simulink model "CDSC"  (R2018b)
settings: Solver=ode45  StartTime=0.0  StopTime=10.0  MaxStep=0.0001  MinStep=0.00001  RelTol=1e-3
libraries: simulink x1, powerlib_meascontrol x1, powerlib x1
settings Model: Creator=lokes  LastModifiedBy=lokes

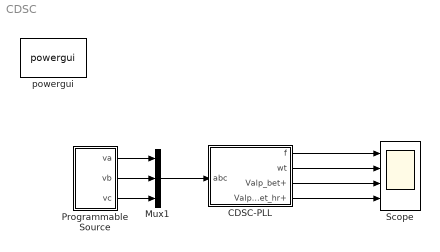
== system CDSC ==
  CDSC-PLL : Subsystem  mask{hr=7}
      mask prompts: hr "Required Component Extraction (hr)"
  Mux1 : Mux  Inputs=3
  Programmable Source : Subsystem  mask(CDSC - PLL){f=50, V=230}
      mask prompts: f "Fundamental grid frequency (f) in Hz"; V "Fundamental grid voltage (V) in RMS volts"
      mask help: Programmable source generates a signal with fundamental and odd harmonic signals upto 13th frequency component.
  Scope : Scope  NumInputPorts=4
  powergui : powerlib/powergui  Priority=1  SimulationMode=Discrete  SampleTime=10e-6  frequency=60  Iterations=50  frequencyindice=60  Pbase=100e6  ErrMax=1e-4  UnitsV=kV  UnitsW=MW  buscounter=0  FunctionMessages=off  echomessages=off  EnableUseOfTLC=off  CurrentSourceSwitches=off  DisableSnubberDevices=off  DisableRonSwitches=off  DisableVfSwitches=off  DisplayEquations=off  SolverType=Tustin/Backward Euler (TBE)  Interpol=off  ExternalGateDelay=off  methode=off  Ts=100  x0status=blocks  SPID=off  SwTol=0  HookPort=off  RestoreLinks=warning  ResistiveCurrentMeasurement=off  Frange=[0:2:500]  Ylog=off  Xlog=on  ShowGrid=off  save=off  variable=ZData  structure=0  ZoomFFT=off  StartTime=0.0  cycles=1  DisplayStyle=1  fundamental=60  FreqAxis=off  MaxFrequency=1000  frequencyindicesteady=1  RmsSteady=1  display=off
  wires:
  Mux1/1 -> CDSC-PLL/1(abc)
  Programmable Source/1(va) -> Mux1/1
  Programmable Source/2(vb) -> Mux1/2
  Programmable Source/3(vc) -> Mux1/3
  CDSC-PLL/1(f) -> Scope/1
  CDSC-PLL/2(wt) -> Scope/2
  CDSC-PLL/3(Valp_bet+) -> Scope/3
  CDSC-PLL/4(Valp_bet_hr+) -> Scope/4

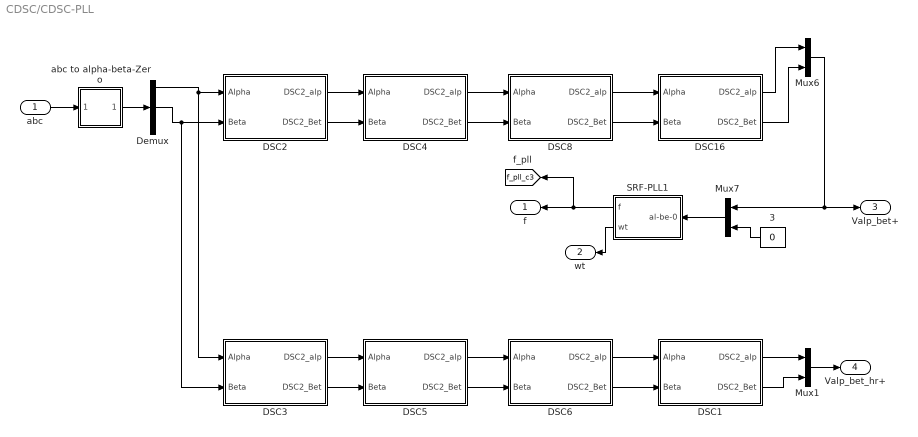
== system CDSC/CDSC-PLL ==
  abc : Inport
  3 : Constant  Value=0
  DSC1 : Subsystem  mask{n=16}
      mask prompts: n "DSC Number (n)"
  DSC16 : Subsystem  mask{n=16}
      mask prompts: n "DSC Number (n)"
  DSC2 : Subsystem  mask{n=2}
      mask prompts: n "DSC Number (n)"
  DSC3 : Subsystem  mask{n=2}
      mask prompts: n "DSC Number (n)"
  DSC4 : Subsystem  mask{n=4}
      mask prompts: n "DSC Number (n)"
  DSC5 : Subsystem  mask{n=4}
      mask prompts: n "DSC Number (n)"
  DSC6 : Subsystem  mask{n=8}
      mask prompts: n "DSC Number (n)"
  DSC8 : Subsystem  mask{n=8}
      mask prompts: n "DSC Number (n)"
  Demux : Demux  Outputs=3
  Mux1 : Mux  Inputs=2
  Mux6 : Mux  Inputs=2
  Mux7 : Mux  Inputs=2
  SRF-PLL1 : Subsystem
  abc to alpha-beta-Zero : Subsystem
      mask Display:
      | plot([0 1], [0,1])
      | text(0.15,0.7,'abc')
      | text(0.55, 0.3,'\alpha\beta0','texmode','on')
  f : Outport
  wt : Outport  Port=2
  Valp_bet+ : Outport  Port=3
  Valp_bet_hr+ : Outport  Port=4
  tag scope: f_pll_c3=global
  wires:
  abc/1 -> abc to alpha-beta-Zero/1(abc)
  abc to alpha-beta-Zero/1(al_be_0) -> Demux/1
  DSC2/1(DSC2_alp) -> DSC4/1(Alpha)
  DSC2/2(DSC2_Bet) -> DSC4/2(Beta)
  DSC4/1(DSC2_alp) -> DSC8/1(Alpha)
  DSC4/2(DSC2_Bet) -> DSC8/2(Beta)
  DSC8/1(DSC2_alp) -> DSC16/1(Alpha)
  DSC8/2(DSC2_Bet) -> DSC16/2(Beta)
  DSC16/1(DSC2_alp) -> Mux6/1
  DSC16/2(DSC2_Bet) -> Mux6/2
  Mux6/1 -> Valp_bet+/1, Mux7/1
  3/1 -> Mux7/2
  Mux7/1 -> SRF-PLL1/1(al-be-0)
  SRF-PLL1/1(f) -> [f_pll_c3], f/1
  SRF-PLL1/2(wt) -> wt/1
  Demux/1 -> DSC3/1(Alpha), DSC2/1(Alpha)
  Demux/2 -> DSC3/2(Beta), DSC2/2(Beta)
  DSC3/1(DSC2_alp) -> DSC5/1(Alpha)
  DSC3/2(DSC2_Bet) -> DSC5/2(Beta)
  DSC5/1(DSC2_alp) -> DSC6/1(Alpha)
  DSC5/2(DSC2_Bet) -> DSC6/2(Beta)
  DSC6/1(DSC2_alp) -> DSC1/1(Alpha)
  DSC6/2(DSC2_Bet) -> DSC1/2(Beta)
  DSC1/1(DSC2_alp) -> Mux1/1
  DSC1/2(DSC2_Bet) -> Mux1/2
  Mux1/1 -> Valp_bet_hr+/1

== system CDSC/Programmable Source ==
  1 : Sin  Amplitude=V*sqrt(2)  Frequency=2*pi*f  Phase=0*pi/2  SampleTime=0
  11 : Sin  Amplitude=V*sqrt(2)/11  Frequency=2*pi*11*f  Phase=0*pi/2  SampleTime=0
  13 : Sin  Amplitude=V*sqrt(2)/13  Frequency=2*pi*13*f  Phase=0*pi/2  SampleTime=0
  5 : Sin  Amplitude=V*sqrt(2)/5  Frequency=2*pi*5*f  Phase=0*pi/2  SampleTime=0
  7 : Sin  Amplitude=V*sqrt(2)/7  Frequency=2*pi*7*f  Phase=0*pi/2  SampleTime=0
  Constant : Constant  Value=2/(3*f)
  Constant1 : Constant  Value=1/(3*f)
  Gain : Gain
  Gain1 : Gain
  Gain2 : Gain
  Sum1 : Sum  Inputs=+++++
  Variable Transport Delay : VariableTransportDelay  VariableDelayType=Variable transport delay  MaximumDelay=10
  Variable Transport Delay1 : VariableTransportDelay  VariableDelayType=Variable transport delay  MaximumDelay=10
  va : Outport
  vb : Outport  Port=2
  vc : Outport  Port=3
  wires:
  Constant1/1 -> Variable Transport Delay1/2
  Constant/1 -> Variable Transport Delay/2
  Variable Transport Delay1/1 -> Gain/1
  Variable Transport Delay/1 -> Gain1/1
  Gain/1 -> vb/1
  Gain1/1 -> vc/1
  Sum1/1 -> Gain2/1
  Gain2/1 -> Variable Transport Delay1/1, Variable Transport Delay/1, va/1
  1/1 -> Sum1/1
  5/1 -> Sum1/2
  7/1 -> Sum1/3
  11/1 -> Sum1/4
  13/1 -> Sum1/5

== system CDSC/CDSC-PLL/DSC1 ==
  Alpha : Inport
  Beta : Inport  Port=2
  DSC_Beta : Subsystem
  DSC_alpha : Subsystem
  DSC2_alp : Outport
  DSC2_Bet : Outport  Port=2
  wires:
  Beta/1 -> DSC_Beta/2(Beta), DSC_alpha/2(Beta)
  Alpha/1 -> DSC_alpha/1(Alpha), DSC_Beta/1(Alpha)
  DSC_Beta/1(Out) -> DSC2_Bet/1
  DSC_alpha/1(Out) -> DSC2_alp/1

== system CDSC/CDSC-PLL/DSC16 ==
  Alpha : Inport
  Beta : Inport  Port=2
  DSC_Beta : Subsystem
  DSC_alpha : Subsystem
  DSC2_alp : Outport
  DSC2_Bet : Outport  Port=2
  wires:
  Beta/1 -> DSC_Beta/2(Beta), DSC_alpha/2(Beta)
  Alpha/1 -> DSC_alpha/1(Alpha), DSC_Beta/1(Alpha)
  DSC_Beta/1(Out) -> DSC2_Bet/1
  DSC_alpha/1(Out) -> DSC2_alp/1

== system CDSC/CDSC-PLL/DSC2 ==
  Alpha : Inport
  Beta : Inport  Port=2
  DSC_Beta : Subsystem
  DSC_alpha : Subsystem
  DSC2_alp : Outport
  DSC2_Bet : Outport  Port=2
  wires:
  DSC_alpha/1(Out) -> DSC2_alp/1
  DSC_Beta/1(Out) -> DSC2_Bet/1
  Alpha/1 -> DSC_Beta/1(Alpha), DSC_alpha/1(Alpha)
  Beta/1 -> DSC_alpha/2(Beta), DSC_Beta/2(Beta)

== system CDSC/CDSC-PLL/DSC3 ==
  Alpha : Inport
  Beta : Inport  Port=2
  DSC_Beta : Subsystem
  DSC_alpha : Subsystem
  DSC2_alp : Outport
  DSC2_Bet : Outport  Port=2
  wires:
  DSC_alpha/1(Out) -> DSC2_alp/1
  DSC_Beta/1(Out) -> DSC2_Bet/1
  Alpha/1 -> DSC_Beta/1(Alpha), DSC_alpha/1(Alpha)
  Beta/1 -> DSC_alpha/2(Beta), DSC_Beta/2(Beta)

== system CDSC/CDSC-PLL/DSC4 ==
  Alpha : Inport
  Beta : Inport  Port=2
  DSC_Beta : Subsystem
  DSC_alpha : Subsystem
  DSC2_alp : Outport
  DSC2_Bet : Outport  Port=2
  wires:
  Beta/1 -> DSC_Beta/2(Beta), DSC_alpha/2(Beta)
  Alpha/1 -> DSC_alpha/1(Alpha), DSC_Beta/1(Alpha)
  DSC_Beta/1(Out) -> DSC2_Bet/1
  DSC_alpha/1(Out) -> DSC2_alp/1

== system CDSC/CDSC-PLL/DSC5 ==
  Alpha : Inport
  Beta : Inport  Port=2
  DSC_Beta : Subsystem
  DSC_alpha : Subsystem
  DSC2_alp : Outport
  DSC2_Bet : Outport  Port=2
  wires:
  Beta/1 -> DSC_Beta/2(Beta), DSC_alpha/2(Beta)
  Alpha/1 -> DSC_alpha/1(Alpha), DSC_Beta/1(Alpha)
  DSC_Beta/1(Out) -> DSC2_Bet/1
  DSC_alpha/1(Out) -> DSC2_alp/1

== system CDSC/CDSC-PLL/DSC6 ==
  Alpha : Inport
  Beta : Inport  Port=2
  DSC_Beta : Subsystem
  DSC_alpha : Subsystem
  DSC2_alp : Outport
  DSC2_Bet : Outport  Port=2
  wires:
  DSC_alpha/1(Out) -> DSC2_alp/1
  DSC_Beta/1(Out) -> DSC2_Bet/1
  Alpha/1 -> DSC_Beta/1(Alpha), DSC_alpha/1(Alpha)
  Beta/1 -> DSC_alpha/2(Beta), DSC_Beta/2(Beta)

== system CDSC/CDSC-PLL/DSC8 ==
  Alpha : Inport
  Beta : Inport  Port=2
  DSC_Beta : Subsystem
  DSC_alpha : Subsystem
  DSC2_alp : Outport
  DSC2_Bet : Outport  Port=2
  wires:
  DSC_alpha/1(Out) -> DSC2_alp/1
  DSC_Beta/1(Out) -> DSC2_Bet/1
  Alpha/1 -> DSC_Beta/1(Alpha), DSC_alpha/1(Alpha)
  Beta/1 -> DSC_alpha/2(Beta), DSC_Beta/2(Beta)

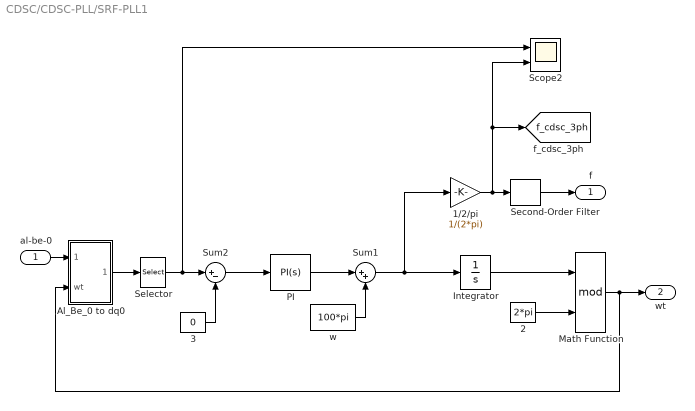
== system CDSC/CDSC-PLL/SRF-PLL1 ==
  al-be-0 : Inport
  1/2/pi : Gain  Gain=1/(2*pi)
  2 : Constant  Value=2*pi
  3 : Constant  Value=0
  Al_Be_0 to dq0 : Subsystem
      mask Display:
      | plot([0 1], [0,1])
      | port_label('input', 1, '\alpha\beta0','texmode','on')
      | port_label('input', 2, 'wt')
      | port_label('output', 1, 'dq0')
  Integrator : Integrator
  Math Function : Math  Operator=mod  SaturateOnIntegerOverflow=on
  "PI " : simulink/Continuous/PID Controller  Controller=PI  Form=Parallel  TimeDomain=Continuous-time  SampleTime=100e-6  IntegratorMethod=Forward Euler  FilterMethod=Forward Euler  ControllerParametersSource=internal  P=10  I=30  D=0  UseFilter=on  N=100  TunerSelectOption=Transfer Function Based (PID Tuner App)  InitialConditionSource=internal  InitialConditionForIntegrator=0  InitialConditionForFilter=0  DifferentiatorICPrevScaledInput=0  ExternalReset=none  TrackingMode=off  Kt=1  LimitOutput=off  UpperSaturationLimit=inf  LowerSaturationLimit=-inf  LinearizeAsGain=on  AntiWindupMode=none  Kb=1  POutMin=[]  POutMax=[]  IOutMin=[]  IOutMax=[]  DOutMin=[]  DOutMax=[]  NOutMin=[]  NOutMax=[]  SumOutMin=[]  SumOutMax=[]  SaturationOutMin=[]  SaturationOutMax=[]  PParamMin=[]  PParamMax=[]  IParamMin=[]  IParamMax=[]  DParamMin=[]  DParamMax=[]  NParamMin=[]  NParamMax=[]  KbParamMin=[]  KbParamMax=[]  KtParamMin=[]  KtParamMax=[]  KbOutMin=[]  KbOutMax=[]  KtOutMin=[]  KtOutMax=[]  IntegratorOutMin=[]  IntegratorOutMax=[]  FilterOutMin=[]  FilterOutMax=[]  SumI1OutMin=[]  SumI1OutMax=[]  SumI2OutMin=[]  SumI2OutMax=[]  SumI3OutMin=[]  SumI3OutMax=[]  SumI4OutMin=[]  SumI4OutMax=[]  SumDOutMin=[]  SumDOutMax=[]  DifferentiatorOutMin=[]  DifferentiatorOutMax=[]  FilterDiffOutCoefMin=[]  FilterDiffOutCoefMax=[]  ReciprocalOutMin=[]  ReciprocalOutMax=[]  SumDenOutMin=[]  SumDenOutMax=[]  SumNumOutMin=[]  SumNumOutMax=[]  DivideOutMin=[]  DivideOutMax=[]  IntegratorContinuousStateAttributes=''  IntegratorStateMustResolveToSignalObject=off  IntegratorRTWStateStorageClass=Auto  FilterContinuousStateAttributes=''  FilterStateMustResolveToSignalObject=off  FilterRTWStateStorageClass=Auto  ParallelPVariant=InternalParameters  IdealPVariant=Disabled  IVariant=InternalParameters  DVariant=Disabled  IntegratorVariant=Continuous  SatVariant=Disabled  AWVariant=Passthrough  PCopyVariant=Disabled  TRVariant=Disabled  FdbkBlocksVariant=Forward  IdealPFdbkVariant=Disabled  SatFdbkVariant=Disabled  DerivativeFilterVariant=Disabled  NVariant=Disabled  NCopyVariant=Disabled_SignalSpec  FilterICVariant=Disabled  IntegratorICVariant=InternalICs  ExternalResetVariant=Disabled  TRSumVariant=Passthrough  SumFdbkVariant=Disabled  SumVariant=Sum_PI
  Scope2 : Scope  NumInputPorts=2
  Second-Order Filter : powerlib_meascontrol/Filters/Second-Order Filter  FilterType=Lowpass  Fo=5  Zeta=0.707  Ts=0  Initialize=off  Vac_Init="[0,  0,  50]"  Vdc_Init=0  PlotResponse=off  FreqRange=[0, 500, 1]
      settings: SourceProductName=Simscape Electrical  SourceProductBaseCode=PS
  Selector : Selector  InputPortWidth=3  IndexOptions=Index vector (dialog)  Indices=1  OutputSizes=1
  Sum1 : Sum  Inputs=|++
  Sum2 : Sum  Inputs=|+-
  w : Constant  Value=100*pi
  f : Outport
  wt : Outport  Port=2
  tag scope: f_cdsc_3ph=global
  wires:
  1/2/pi/1 -> Second-Order Filter/1, [f_cdsc_3ph], Scope2/2
  Math Function/1 -> Al_Be_0 to dq0/2(wt), wt/1
  Integrator/1 -> Math Function/1
  2/1 -> Math Function/2
  Sum1/1 -> Integrator/1, 1/2/pi/1
  w/1 -> Sum1/2
  "PI "/1 -> Sum1/1
  Sum2/1 -> "PI "/1
  al-be-0/1 -> Al_Be_0 to dq0/1(Al_Be_0)
  3/1 -> Sum2/2
  Al_Be_0 to dq0/1(dq0) -> Selector/1
  Selector/1 -> Sum2/1, Scope2/1
  Second-Order Filter/1 -> f/1

== system CDSC/CDSC-PLL/abc to alpha-beta-Zero ==
  abc : Inport
  Gain1 : Gain  Gain=(2/3)  SaturateOnIntegerOverflow=on  OutDataTypeStr=Inherit: Same as input  ParamDataTypeStr=Inherit: Same as input
  Gain3 : Gain  Gain="[ 1   -1/2   -1/2; 0   sqrt(3)/2   -sqrt(3)/2; 1/(2)  1/(2)  1/(2) ]"  Multiplication=Matrix(K*u) (u vector)  SaturateOnIntegerOverflow=on  OutDataTypeStr=Inherit: Same as input  ParamDataTypeStr=Inherit: Same as input
  al_be_0 : Outport
  wires:
  Gain3/1 -> Gain1/1
  Gain1/1 -> al_be_0/1
  abc/1 -> Gain3/1

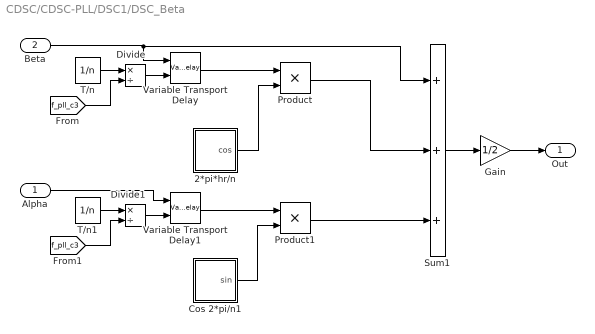
== system CDSC/CDSC-PLL/DSC1/DSC_Beta ==
  Alpha : Inport
  Beta : Inport  Port=2
  2*pi*hr/n : Subsystem
  Cos 2*pi/n1 : Subsystem
  Divide : Product  Inputs=*/
  Divide1 : Product  Inputs=*/
  Gain : Gain  Gain=1/2
  Product : Product
  Product1 : Product
  Sum1 : Sum  Inputs=+++
  T/n : Constant  Value=1/n
  T/n1 : Constant  Value=1/n
  Variable Transport Delay : VariableTransportDelay  VariableDelayType=Variable transport delay  MaximumDelay=10
  Variable Transport Delay1 : VariableTransportDelay  VariableDelayType=Variable transport delay  MaximumDelay=10
  Out : Outport
  wires:
  Gain/1 -> Out/1
  Sum1/1 -> Gain/1
  Beta/1 -> Variable Transport Delay/1, Sum1/1
  Alpha/1 -> Variable Transport Delay1/1
  2*pi*hr/n/1(cos) -> Product/2
  Product/1 -> Sum1/2
  Variable Transport Delay/1 -> Product/1
  Variable Transport Delay1/1 -> Product1/1
  Product1/1 -> Sum1/3
  Cos 2*pi/n1/1(sin) -> Product1/2
  T/n/1 -> Divide/1
  Divide/1 -> Variable Transport Delay/2
  [f_pll_c3] -> Divide/2
  T/n1/1 -> Divide1/1
  Divide1/1 -> Variable Transport Delay1/2
  [f_pll_c3] -> Divide1/2

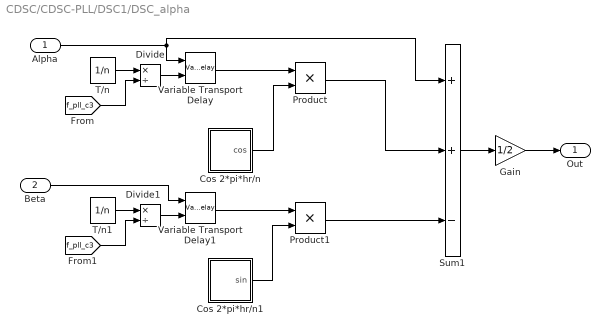
== system CDSC/CDSC-PLL/DSC1/DSC_alpha ==
  Alpha : Inport
  Beta : Inport  Port=2
  Cos 2*pi*hr/n : Subsystem
  Cos 2*pi*hr/n1 : Subsystem
  Divide : Product  Inputs=*/
  Divide1 : Product  Inputs=*/
  Gain : Gain  Gain=1/2
  Product : Product
  Product1 : Product
  Sum1 : Sum  Inputs=++-
  T/n : Constant  Value=1/n
  T/n1 : Constant  Value=1/n
  Variable Transport Delay : VariableTransportDelay  VariableDelayType=Variable transport delay  MaximumDelay=10
  Variable Transport Delay1 : VariableTransportDelay  VariableDelayType=Variable transport delay  MaximumDelay=10
  Out : Outport
  wires:
  Sum1/1 -> Gain/1
  Gain/1 -> Out/1
  Cos 2*pi*hr/n1/1(sin) -> Product1/2
  Beta/1 -> Variable Transport Delay1/1
  Product1/1 -> Sum1/3
  Variable Transport Delay1/1 -> Product1/1
  Alpha/1 -> Variable Transport Delay/1, Sum1/1
  Variable Transport Delay/1 -> Product/1
  Product/1 -> Sum1/2
  Cos 2*pi*hr/n/1(cos) -> Product/2
  T/n/1 -> Divide/1
  Divide/1 -> Variable Transport Delay/2
  [f_pll_c3] -> Divide/2
  T/n1/1 -> Divide1/1
  Divide1/1 -> Variable Transport Delay1/2
  [f_pll_c3] -> Divide1/2

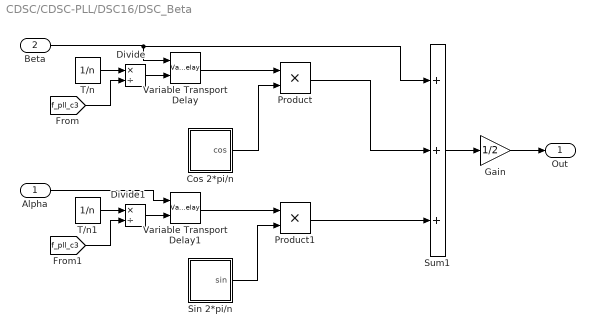
== system CDSC/CDSC-PLL/DSC16/DSC_Beta ==
  Alpha : Inport
  Beta : Inport  Port=2
  Cos 2*pi/n : Subsystem
  Divide : Product  Inputs=*/
  Divide1 : Product  Inputs=*/
  Gain : Gain  Gain=1/2
  Product : Product
  Product1 : Product
  Sin 2*pi/n : Subsystem
  Sum1 : Sum  Inputs=+++
  T/n : Constant  Value=1/n
  T/n1 : Constant  Value=1/n
  Variable Transport Delay : VariableTransportDelay  VariableDelayType=Variable transport delay  MaximumDelay=10
  Variable Transport Delay1 : VariableTransportDelay  VariableDelayType=Variable transport delay  MaximumDelay=10
  Out : Outport
  wires:
  Gain/1 -> Out/1
  Sum1/1 -> Gain/1
  Beta/1 -> Variable Transport Delay/1, Sum1/1
  Alpha/1 -> Variable Transport Delay1/1
  Cos 2*pi/n/1(cos) -> Product/2
  Product/1 -> Sum1/2
  Variable Transport Delay/1 -> Product/1
  Variable Transport Delay1/1 -> Product1/1
  Product1/1 -> Sum1/3
  Sin 2*pi/n/1(sin) -> Product1/2
  T/n/1 -> Divide/1
  Divide/1 -> Variable Transport Delay/2
  [f_pll_c3] -> Divide/2
  T/n1/1 -> Divide1/1
  Divide1/1 -> Variable Transport Delay1/2
  [f_pll_c3] -> Divide1/2

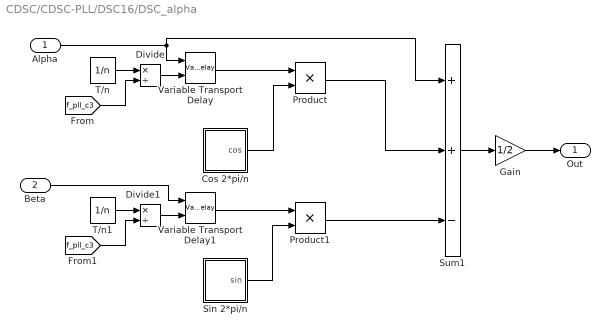
== system CDSC/CDSC-PLL/DSC16/DSC_alpha ==
  Alpha : Inport
  Beta : Inport  Port=2
  Cos 2*pi/n : Subsystem
  Divide : Product  Inputs=*/
  Divide1 : Product  Inputs=*/
  Gain : Gain  Gain=1/2
  Product : Product
  Product1 : Product
  Sin 2*pi/n : Subsystem
  Sum1 : Sum  Inputs=++-
  T/n : Constant  Value=1/n
  T/n1 : Constant  Value=1/n
  Variable Transport Delay : VariableTransportDelay  VariableDelayType=Variable transport delay  MaximumDelay=10
  Variable Transport Delay1 : VariableTransportDelay  VariableDelayType=Variable transport delay  MaximumDelay=10
  Out : Outport
  wires:
  Sum1/1 -> Gain/1
  Gain/1 -> Out/1
  Sin 2*pi/n/1(sin) -> Product1/2
  Beta/1 -> Variable Transport Delay1/1
  Product1/1 -> Sum1/3
  Variable Transport Delay1/1 -> Product1/1
  Alpha/1 -> Variable Transport Delay/1, Sum1/1
  Variable Transport Delay/1 -> Product/1
  Product/1 -> Sum1/2
  Cos 2*pi/n/1(cos) -> Product/2
  T/n/1 -> Divide/1
  Divide/1 -> Variable Transport Delay/2
  [f_pll_c3] -> Divide/2
  T/n1/1 -> Divide1/1
  Divide1/1 -> Variable Transport Delay1/2
  [f_pll_c3] -> Divide1/2

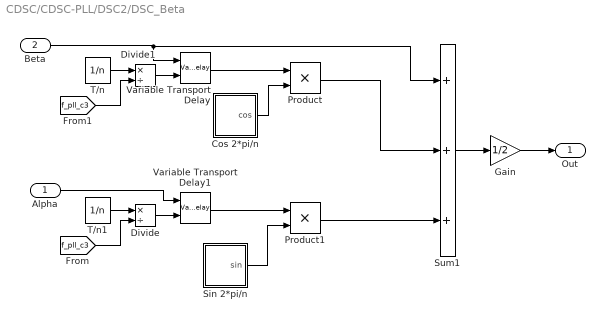
== system CDSC/CDSC-PLL/DSC2/DSC_Beta ==
  Alpha : Inport
  Beta : Inport  Port=2
  Cos 2*pi/n : Subsystem
  Divide : Product  Inputs=*/
  Divide1 : Product  Inputs=*/
  Gain : Gain  Gain=1/2
  Product : Product
  Product1 : Product
  Sin 2*pi/n : Subsystem
  Sum1 : Sum  Inputs=+++
  T/n : Constant  Value=1/n
  T/n1 : Constant  Value=1/n
  Variable Transport Delay : VariableTransportDelay  VariableDelayType=Variable transport delay  MaximumDelay=10
  Variable Transport Delay1 : VariableTransportDelay  VariableDelayType=Variable transport delay  MaximumDelay=10
  Out : Outport
  wires:
  Sin 2*pi/n/1(sin) -> Product1/2
  Product1/1 -> Sum1/3
  Variable Transport Delay1/1 -> Product1/1
  Variable Transport Delay/1 -> Product/1
  Product/1 -> Sum1/2
  Cos 2*pi/n/1(cos) -> Product/2
  Alpha/1 -> Variable Transport Delay1/1
  Beta/1 -> Sum1/1, Variable Transport Delay/1
  Sum1/1 -> Gain/1
  Gain/1 -> Out/1
  T/n1/1 -> Divide/1
  Divide/1 -> Variable Transport Delay1/2
  [f_pll_c3] -> Divide/2
  T/n/1 -> Divide1/1
  Divide1/1 -> Variable Transport Delay/2
  [f_pll_c3] -> Divide1/2

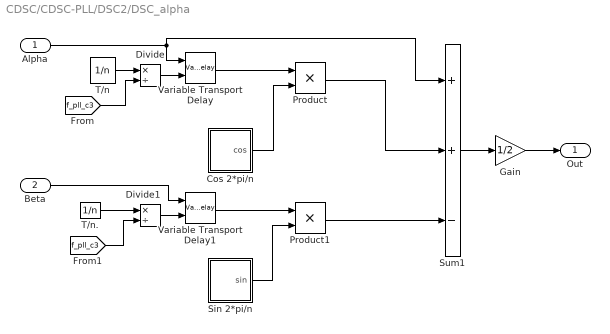
== system CDSC/CDSC-PLL/DSC2/DSC_alpha ==
  Alpha : Inport
  Beta : Inport  Port=2
  Cos 2*pi/n : Subsystem
  Divide : Product  Inputs=*/
  Divide1 : Product  Inputs=*/
  Gain : Gain  Gain=1/2
  Product : Product
  Product1 : Product
  Sin 2*pi/n : Subsystem
  Sum1 : Sum  Inputs=++-
  T/n : Constant  Value=1/n
  T/n. : Constant  Value=1/n
  Variable Transport Delay : VariableTransportDelay  VariableDelayType=Variable transport delay  MaximumDelay=10
  Variable Transport Delay1 : VariableTransportDelay  VariableDelayType=Variable transport delay  MaximumDelay=10
  Out : Outport
  wires:
  Cos 2*pi/n/1(cos) -> Product/2
  Product/1 -> Sum1/2
  Variable Transport Delay/1 -> Product/1
  Alpha/1 -> Variable Transport Delay/1, Sum1/1
  Variable Transport Delay1/1 -> Product1/1
  Product1/1 -> Sum1/3
  Beta/1 -> Variable Transport Delay1/1
  Sin 2*pi/n/1(sin) -> Product1/2
  Gain/1 -> Out/1
  Sum1/1 -> Gain/1
  T/n/1 -> Divide/1
  Divide/1 -> Variable Transport Delay/2
  [f_pll_c3] -> Divide/2
  Divide1/1 -> Variable Transport Delay1/2
  T/n./1 -> Divide1/1
  [f_pll_c3] -> Divide1/2

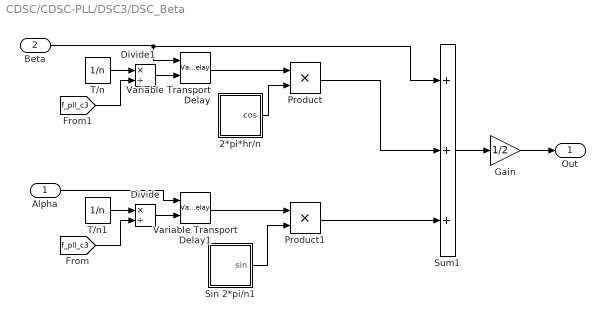
== system CDSC/CDSC-PLL/DSC3/DSC_Beta ==
  Alpha : Inport
  Beta : Inport  Port=2
  2*pi*hr/n : Subsystem
  Divide : Product  Inputs=*/
  Divide1 : Product  Inputs=*/
  Gain : Gain  Gain=1/2
  Product : Product
  Product1 : Product
  Sin 2*pi/n1 : Subsystem
  Sum1 : Sum  Inputs=+++
  T/n : Constant  Value=1/n
  T/n1 : Constant  Value=1/n
  Variable Transport Delay : VariableTransportDelay  VariableDelayType=Variable transport delay  MaximumDelay=10
  Variable Transport Delay1 : VariableTransportDelay  VariableDelayType=Variable transport delay  MaximumDelay=10
  Out : Outport
  wires:
  Sin 2*pi/n1/1(sin) -> Product1/2
  Product1/1 -> Sum1/3
  Variable Transport Delay1/1 -> Product1/1
  Variable Transport Delay/1 -> Product/1
  Product/1 -> Sum1/2
  2*pi*hr/n/1(cos) -> Product/2
  Alpha/1 -> Variable Transport Delay1/1
  Beta/1 -> Sum1/1, Variable Transport Delay/1
  Sum1/1 -> Gain/1
  Gain/1 -> Out/1
  T/n1/1 -> Divide/1
  Divide/1 -> Variable Transport Delay1/2
  [f_pll_c3] -> Divide/2
  T/n/1 -> Divide1/1
  Divide1/1 -> Variable Transport Delay/2
  [f_pll_c3] -> Divide1/2

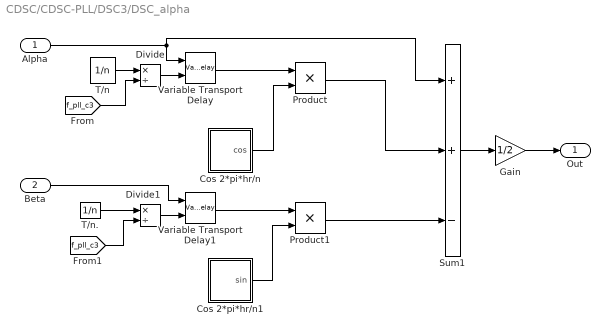
== system CDSC/CDSC-PLL/DSC3/DSC_alpha ==
  Alpha : Inport
  Beta : Inport  Port=2
  Cos 2*pi*hr/n : Subsystem
  Cos 2*pi*hr/n1 : Subsystem
  Divide : Product  Inputs=*/
  Divide1 : Product  Inputs=*/
  Gain : Gain  Gain=1/2
  Product : Product
  Product1 : Product
  Sum1 : Sum  Inputs=++-
  T/n : Constant  Value=1/n
  T/n. : Constant  Value=1/n
  Variable Transport Delay : VariableTransportDelay  VariableDelayType=Variable transport delay  MaximumDelay=10
  Variable Transport Delay1 : VariableTransportDelay  VariableDelayType=Variable transport delay  MaximumDelay=10
  Out : Outport
  wires:
  Cos 2*pi*hr/n/1(cos) -> Product/2
  Product/1 -> Sum1/2
  Variable Transport Delay/1 -> Product/1
  Alpha/1 -> Variable Transport Delay/1, Sum1/1
  Variable Transport Delay1/1 -> Product1/1
  Product1/1 -> Sum1/3
  Beta/1 -> Variable Transport Delay1/1
  Cos 2*pi*hr/n1/1(sin) -> Product1/2
  Gain/1 -> Out/1
  Sum1/1 -> Gain/1
  T/n/1 -> Divide/1
  Divide/1 -> Variable Transport Delay/2
  [f_pll_c3] -> Divide/2
  Divide1/1 -> Variable Transport Delay1/2
  T/n./1 -> Divide1/1
  [f_pll_c3] -> Divide1/2

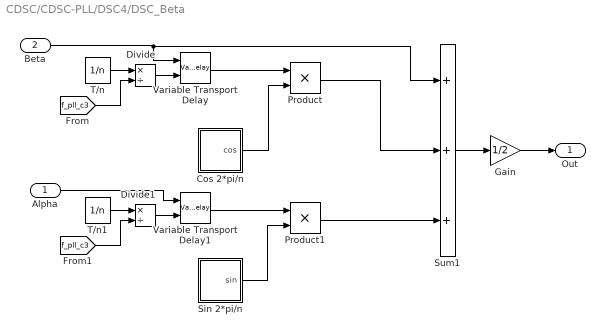
== system CDSC/CDSC-PLL/DSC4/DSC_Beta ==
  Alpha : Inport
  Beta : Inport  Port=2
  Cos 2*pi/n : Subsystem
  Divide : Product  Inputs=*/
  Divide1 : Product  Inputs=*/
  Gain : Gain  Gain=1/2
  Product : Product
  Product1 : Product
  Sin 2*pi/n : Subsystem
  Sum1 : Sum  Inputs=+++
  T/n : Constant  Value=1/n
  T/n1 : Constant  Value=1/n
  Variable Transport Delay : VariableTransportDelay  VariableDelayType=Variable transport delay  MaximumDelay=10
  Variable Transport Delay1 : VariableTransportDelay  VariableDelayType=Variable transport delay  MaximumDelay=10
  Out : Outport
  wires:
  Gain/1 -> Out/1
  Sum1/1 -> Gain/1
  Beta/1 -> Variable Transport Delay/1, Sum1/1
  Alpha/1 -> Variable Transport Delay1/1
  Cos 2*pi/n/1(cos) -> Product/2
  Product/1 -> Sum1/2
  Variable Transport Delay/1 -> Product/1
  Variable Transport Delay1/1 -> Product1/1
  Product1/1 -> Sum1/3
  Sin 2*pi/n/1(sin) -> Product1/2
  T/n/1 -> Divide/1
  Divide/1 -> Variable Transport Delay/2
  [f_pll_c3] -> Divide/2
  T/n1/1 -> Divide1/1
  Divide1/1 -> Variable Transport Delay1/2
  [f_pll_c3] -> Divide1/2

== system CDSC/CDSC-PLL/DSC4/DSC_alpha ==
  Alpha : Inport
  Beta : Inport  Port=2
  Cos 2*pi/n : Subsystem
  Divide : Product  Inputs=*/
  Divide1 : Product  Inputs=*/
  Gain : Gain  Gain=1/2
  Product : Product
  Product1 : Product
  Sin 2*pi/n : Subsystem
  Sum1 : Sum  Inputs=++-
  T/n : Constant  Value=1/n
  T/n1 : Constant  Value=1/n
  Variable Transport Delay : VariableTransportDelay  VariableDelayType=Variable transport delay  MaximumDelay=10
  Variable Transport Delay1 : VariableTransportDelay  VariableDelayType=Variable transport delay  MaximumDelay=10
  Out : Outport
  wires:
  Sum1/1 -> Gain/1
  Gain/1 -> Out/1
  Sin 2*pi/n/1(sin) -> Product1/2
  Beta/1 -> Variable Transport Delay1/1
  Product1/1 -> Sum1/3
  Variable Transport Delay1/1 -> Product1/1
  Alpha/1 -> Variable Transport Delay/1, Sum1/1
  Variable Transport Delay/1 -> Product/1
  Product/1 -> Sum1/2
  Cos 2*pi/n/1(cos) -> Product/2
  T/n1/1 -> Divide/1
  Divide/1 -> Variable Transport Delay1/2
  [f_pll_c3] -> Divide/2
  T/n/1 -> Divide1/1
  Divide1/1 -> Variable Transport Delay/2
  [f_pll_c3] -> Divide1/2

== system CDSC/CDSC-PLL/DSC5/DSC_Beta ==
  Alpha : Inport
  Beta : Inport  Port=2
  2*pi*hr/n : Subsystem
  Cos 2*pi/n1 : Subsystem
  Divide : Product  Inputs=*/
  Divide1 : Product  Inputs=*/
  Gain : Gain  Gain=1/2
  Product : Product
  Product1 : Product
  Sum1 : Sum  Inputs=+++
  T/n : Constant  Value=1/n
  T/n1 : Constant  Value=1/n
  Variable Transport Delay : VariableTransportDelay  VariableDelayType=Variable transport delay  MaximumDelay=10
  Variable Transport Delay1 : VariableTransportDelay  VariableDelayType=Variable transport delay  MaximumDelay=10
  Out : Outport
  wires:
  Gain/1 -> Out/1
  Sum1/1 -> Gain/1
  Beta/1 -> Variable Transport Delay/1, Sum1/1
  Alpha/1 -> Variable Transport Delay1/1
  2*pi*hr/n/1(cos) -> Product/2
  Product/1 -> Sum1/2
  Variable Transport Delay/1 -> Product/1
  Variable Transport Delay1/1 -> Product1/1
  Product1/1 -> Sum1/3
  Cos 2*pi/n1/1(sin) -> Product1/2
  T/n/1 -> Divide/1
  Divide/1 -> Variable Transport Delay/2
  [f_pll_c3] -> Divide/2
  T/n1/1 -> Divide1/1
  Divide1/1 -> Variable Transport Delay1/2
  [f_pll_c3] -> Divide1/2

== system CDSC/CDSC-PLL/DSC5/DSC_alpha ==
  Alpha : Inport
  Beta : Inport  Port=2
  Cos 2*pi*hr/n : Subsystem
  Cos 2*pi*hr/n1 : Subsystem
  Divide : Product  Inputs=*/
  Divide1 : Product  Inputs=*/
  Gain : Gain  Gain=1/2
  Product : Product
  Product1 : Product
  Sum1 : Sum  Inputs=++-
  T/n : Constant  Value=1/n
  T/n1 : Constant  Value=1/n
  Variable Transport Delay : VariableTransportDelay  VariableDelayType=Variable transport delay  MaximumDelay=10
  Variable Transport Delay1 : VariableTransportDelay  VariableDelayType=Variable transport delay  MaximumDelay=10
  Out : Outport
  wires:
  Sum1/1 -> Gain/1
  Gain/1 -> Out/1
  Cos 2*pi*hr/n1/1(sin) -> Product1/2
  Beta/1 -> Variable Transport Delay1/1
  Product1/1 -> Sum1/3
  Variable Transport Delay1/1 -> Product1/1
  Alpha/1 -> Variable Transport Delay/1, Sum1/1
  Variable Transport Delay/1 -> Product/1
  Product/1 -> Sum1/2
  Cos 2*pi*hr/n/1(cos) -> Product/2
  T/n1/1 -> Divide/1
  Divide/1 -> Variable Transport Delay1/2
  [f_pll_c3] -> Divide/2
  T/n/1 -> Divide1/1
  Divide1/1 -> Variable Transport Delay/2
  [f_pll_c3] -> Divide1/2

== system CDSC/CDSC-PLL/DSC6/DSC_Beta ==
  Alpha : Inport
  Beta : Inport  Port=2
  2*pi*hr/n : Subsystem
  Cos 2*pi/n1 : Subsystem
  Divide : Product  Inputs=*/
  Divide1 : Product  Inputs=*/
  Gain : Gain  Gain=1/2
  Product : Product
  Product1 : Product
  Sum1 : Sum  Inputs=+++
  T/n : Constant  Value=1/n
  T/n1 : Constant  Value=1/n
  Variable Transport Delay : VariableTransportDelay  VariableDelayType=Variable transport delay  MaximumDelay=10
  Variable Transport Delay1 : VariableTransportDelay  VariableDelayType=Variable transport delay  MaximumDelay=10
  Out : Outport
  wires:
  Cos 2*pi/n1/1(sin) -> Product1/2
  Product1/1 -> Sum1/3
  Variable Transport Delay1/1 -> Product1/1
  Variable Transport Delay/1 -> Product/1
  Product/1 -> Sum1/2
  2*pi*hr/n/1(cos) -> Product/2
  Alpha/1 -> Variable Transport Delay1/1
  Beta/1 -> Sum1/1, Variable Transport Delay/1
  Sum1/1 -> Gain/1
  Gain/1 -> Out/1
  T/n/1 -> Divide/1
  Divide/1 -> Variable Transport Delay/2
  [f_pll_c3] -> Divide/2
  T/n1/1 -> Divide1/1
  Divide1/1 -> Variable Transport Delay1/2
  [f_pll_c3] -> Divide1/2

== system CDSC/CDSC-PLL/DSC6/DSC_alpha ==
  Alpha : Inport
  Beta : Inport  Port=2
  Cos 2*pi*hr/n : Subsystem
  Cos 2*pi*hr/n1 : Subsystem
  Divide : Product  Inputs=*/
  Divide1 : Product  Inputs=*/
  Gain : Gain  Gain=1/2
  Product : Product
  Product1 : Product
  Sum1 : Sum  Inputs=++-
  T/n : Constant  Value=1/n
  T/n1 : Constant  Value=1/n
  Variable Transport Delay : VariableTransportDelay  VariableDelayType=Variable transport delay  MaximumDelay=10
  Variable Transport Delay1 : VariableTransportDelay  VariableDelayType=Variable transport delay  MaximumDelay=10
  Out : Outport
  wires:
  Cos 2*pi*hr/n/1(cos) -> Product/2
  Product/1 -> Sum1/2
  Variable Transport Delay/1 -> Product/1
  Alpha/1 -> Variable Transport Delay/1, Sum1/1
  Variable Transport Delay1/1 -> Product1/1
  Product1/1 -> Sum1/3
  Beta/1 -> Variable Transport Delay1/1
  Cos 2*pi*hr/n1/1(sin) -> Product1/2
  Gain/1 -> Out/1
  Sum1/1 -> Gain/1
  T/n/1 -> Divide/1
  Divide/1 -> Variable Transport Delay/2
  [f_pll_c3] -> Divide/2
  T/n1/1 -> Divide1/1
  Divide1/1 -> Variable Transport Delay1/2
  [f_pll_c3] -> Divide1/2

== system CDSC/CDSC-PLL/DSC8/DSC_Beta ==
  Alpha : Inport
  Beta : Inport  Port=2
  Cos 2*pi/n : Subsystem
  Divide : Product  Inputs=*/
  Divide1 : Product  Inputs=*/
  Gain : Gain  Gain=1/2
  Product : Product
  Product1 : Product
  Sin 2*pi/n : Subsystem
  Sum1 : Sum  Inputs=+++
  T/n : Constant  Value=1/n
  T/n1 : Constant  Value=1/n
  Variable Transport Delay : VariableTransportDelay  VariableDelayType=Variable transport delay  MaximumDelay=10
  Variable Transport Delay1 : VariableTransportDelay  VariableDelayType=Variable transport delay  MaximumDelay=10
  Out : Outport
  wires:
  Sin 2*pi/n/1(sin) -> Product1/2
  Product1/1 -> Sum1/3
  Variable Transport Delay1/1 -> Product1/1
  Variable Transport Delay/1 -> Product/1
  Product/1 -> Sum1/2
  Cos 2*pi/n/1(cos) -> Product/2
  Alpha/1 -> Variable Transport Delay1/1
  Beta/1 -> Sum1/1, Variable Transport Delay/1
  Sum1/1 -> Gain/1
  Gain/1 -> Out/1
  T/n/1 -> Divide/1
  Divide/1 -> Variable Transport Delay/2
  [f_pll_c3] -> Divide/2
  T/n1/1 -> Divide1/1
  Divide1/1 -> Variable Transport Delay1/2
  [f_pll_c3] -> Divide1/2

== system CDSC/CDSC-PLL/DSC8/DSC_alpha ==
  Alpha : Inport
  Beta : Inport  Port=2
  Cos 2*pi/n : Subsystem
  Divide : Product  Inputs=*/
  Divide1 : Product  Inputs=*/
  Gain : Gain  Gain=1/2
  Product : Product
  Product1 : Product
  Sin 2*pi/n : Subsystem
  Sum1 : Sum  Inputs=++-
  T/n : Constant  Value=1/n
  T/n1 : Constant  Value=1/n
  Variable Transport Delay : VariableTransportDelay  VariableDelayType=Variable transport delay  MaximumDelay=10
  Variable Transport Delay1 : VariableTransportDelay  VariableDelayType=Variable transport delay  MaximumDelay=10
  Out : Outport
  wires:
  Cos 2*pi/n/1(cos) -> Product/2
  Product/1 -> Sum1/2
  Variable Transport Delay/1 -> Product/1
  Alpha/1 -> Variable Transport Delay/1, Sum1/1
  Variable Transport Delay1/1 -> Product1/1
  Product1/1 -> Sum1/3
  Beta/1 -> Variable Transport Delay1/1
  Sin 2*pi/n/1(sin) -> Product1/2
  Gain/1 -> Out/1
  Sum1/1 -> Gain/1
  T/n/1 -> Divide/1
  Divide/1 -> Variable Transport Delay/2
  [f_pll_c3] -> Divide/2
  T/n1/1 -> Divide1/1
  Divide1/1 -> Variable Transport Delay1/2
  [f_pll_c3] -> Divide1/2

== system CDSC/CDSC-PLL/SRF-PLL1/Al_Be_0 to dq0 ==
  Al_Be_0 : Inport
  wt : Inport  Port=2
  Fcn : Fcn  Expr=u[1]*cos(u[4]) + u[2]*sin(u[4])
  Fcn1 : Fcn  Expr=-u[1]*sin(u[4]) + u[2]*cos(u[4])
  Fcn2 : Fcn  Expr=u[3]
  Mux1 : Mux  Inputs=[3 1]
  Mux2 : Mux  Inputs=3
  dq0 : Outport
  wires:
  Mux1/1 -> Fcn/1, Fcn2/1, Fcn1/1
  Fcn1/1 -> Mux2/2
  wt/1 -> Mux1/2
  Mux2/1 -> dq0/1
  Al_Be_0/1 -> Mux1/1
  Fcn2/1 -> Mux2/3
  Fcn/1 -> Mux2/1

== system CDSC/CDSC-PLL/DSC1/DSC_Beta/2*pi*hr//n ==
  note: 2*pi*hr/n
  Constant : Constant  Value=2*pi*hr/n
  Trigonometric Function : Trigonometry  Operator=cos
  cos : Outport
  wires:
  Constant/1 -> Trigonometric Function/1
  Trigonometric Function/1 -> cos/1

== system CDSC/CDSC-PLL/DSC1/DSC_Beta/Cos 2*pi//n1 ==
  note: 2*pi*hr/n
  Constant : Constant  Value=2*pi*hr/n
  Trigonometric Function : Trigonometry
  sin : Outport
  wires:
  Constant/1 -> Trigonometric Function/1
  Trigonometric Function/1 -> sin/1

== system CDSC/CDSC-PLL/DSC1/DSC_alpha/Cos 2*pi*hr//n ==
  note: 2*pi*hr/n
  Constant : Constant  Value=2*pi*hr/n
  Trigonometric Function : Trigonometry  Operator=cos
  cos : Outport
  wires:
  Constant/1 -> Trigonometric Function/1
  Trigonometric Function/1 -> cos/1

== system CDSC/CDSC-PLL/DSC1/DSC_alpha/Cos 2*pi*hr//n1 ==
  note: 2*pi*hr/n
  Constant : Constant  Value=2*pi*hr/n
  Trigonometric Function : Trigonometry
  sin : Outport
  wires:
  Constant/1 -> Trigonometric Function/1
  Trigonometric Function/1 -> sin/1

== system CDSC/CDSC-PLL/DSC16/DSC_Beta/Cos 2*pi//n ==
  note: 2*pi*hr/n
  Constant : Constant  Value=2*pi/n
  Trigonometric Function : Trigonometry  Operator=cos
  cos : Outport
  wires:
  Trigonometric Function/1 -> cos/1
  Constant/1 -> Trigonometric Function/1

== system CDSC/CDSC-PLL/DSC16/DSC_Beta/Sin 2*pi//n ==
  note: 2*pi/n
  Constant : Constant  Value=2*pi/n
  Trigonometric Function : Trigonometry
  sin : Outport
  wires:
  Trigonometric Function/1 -> sin/1
  Constant/1 -> Trigonometric Function/1

== system CDSC/CDSC-PLL/DSC16/DSC_alpha/Cos 2*pi//n ==
  note: 2*pi*hr/n
  Constant : Constant  Value=2*pi/n
  Trigonometric Function : Trigonometry  Operator=cos
  cos : Outport
  wires:
  Trigonometric Function/1 -> cos/1
  Constant/1 -> Trigonometric Function/1

== system CDSC/CDSC-PLL/DSC16/DSC_alpha/Sin 2*pi//n ==
  note: 2*pi/n
  Constant : Constant  Value=2*pi/n
  Trigonometric Function : Trigonometry
  sin : Outport
  wires:
  Trigonometric Function/1 -> sin/1
  Constant/1 -> Trigonometric Function/1

== system CDSC/CDSC-PLL/DSC2/DSC_Beta/Cos 2*pi//n ==
  note: 2*pi*hr/n
  Constant : Constant  Value=2*pi/n
  Trigonometric Function : Trigonometry  Operator=cos
  cos : Outport
  wires:
  Trigonometric Function/1 -> cos/1
  Constant/1 -> Trigonometric Function/1

== system CDSC/CDSC-PLL/DSC2/DSC_Beta/Sin 2*pi//n ==
  note: 2*pi/n
  Constant : Constant  Value=2*pi/n
  Trigonometric Function : Trigonometry
  sin : Outport
  wires:
  Trigonometric Function/1 -> sin/1
  Constant/1 -> Trigonometric Function/1

== system CDSC/CDSC-PLL/DSC2/DSC_alpha/Cos 2*pi//n ==
  note: 2*pi*hr/n
  Constant : Constant  Value=2*pi/n
  Trigonometric Function : Trigonometry  Operator=cos
  cos : Outport
  wires:
  Trigonometric Function/1 -> cos/1
  Constant/1 -> Trigonometric Function/1

== system CDSC/CDSC-PLL/DSC2/DSC_alpha/Sin 2*pi//n ==
  note: 2*pi/n
  Constant : Constant  Value=2*pi/n
  Trigonometric Function : Trigonometry
  sin : Outport
  wires:
  Trigonometric Function/1 -> sin/1
  Constant/1 -> Trigonometric Function/1

== system CDSC/CDSC-PLL/DSC3/DSC_Beta/2*pi*hr//n ==
  note: 2*pi*hr/n
  Constant : Constant  Value=2*pi*hr/n
  Trigonometric Function : Trigonometry  Operator=cos
  cos : Outport
  wires:
  Trigonometric Function/1 -> cos/1
  Constant/1 -> Trigonometric Function/1

== system CDSC/CDSC-PLL/DSC3/DSC_Beta/Sin 2*pi//n1 ==
  note: 2*pi*hr/n
  Constant : Constant  Value=2*pi*hr/n
  Trigonometric Function : Trigonometry
  sin : Outport
  wires:
  Trigonometric Function/1 -> sin/1
  Constant/1 -> Trigonometric Function/1

== system CDSC/CDSC-PLL/DSC3/DSC_alpha/Cos 2*pi*hr//n ==
  note: 2*pi*hr/n
  Constant : Constant  Value=2*pi*hr/n
  Trigonometric Function : Trigonometry  Operator=cos
  cos : Outport
  wires:
  Trigonometric Function/1 -> cos/1
  Constant/1 -> Trigonometric Function/1

== system CDSC/CDSC-PLL/DSC3/DSC_alpha/Cos 2*pi*hr//n1 ==
  note: 2*pi*hr/n
  Constant : Constant  Value=2*pi*hr/n
  Trigonometric Function : Trigonometry
  sin : Outport
  wires:
  Trigonometric Function/1 -> sin/1
  Constant/1 -> Trigonometric Function/1

== system CDSC/CDSC-PLL/DSC4/DSC_Beta/Cos 2*pi//n ==
  note: 2*pi*hr/n
  Constant : Constant  Value=2*pi/n
  Trigonometric Function : Trigonometry  Operator=cos
  cos : Outport
  wires:
  Trigonometric Function/1 -> cos/1
  Constant/1 -> Trigonometric Function/1

== system CDSC/CDSC-PLL/DSC4/DSC_Beta/Sin 2*pi//n ==
  note: 2*pi/n
  Constant : Constant  Value=2*pi/n
  Trigonometric Function : Trigonometry
  sin : Outport
  wires:
  Trigonometric Function/1 -> sin/1
  Constant/1 -> Trigonometric Function/1

== system CDSC/CDSC-PLL/DSC4/DSC_alpha/Cos 2*pi//n ==
  note: 2*pi*hr/n
  Constant : Constant  Value=2*pi/n
  Trigonometric Function : Trigonometry  Operator=cos
  cos : Outport
  wires:
  Trigonometric Function/1 -> cos/1
  Constant/1 -> Trigonometric Function/1

== system CDSC/CDSC-PLL/DSC4/DSC_alpha/Sin 2*pi//n ==
  note: 2*pi/n
  Constant : Constant  Value=2*pi/n
  Trigonometric Function : Trigonometry
  sin : Outport
  wires:
  Trigonometric Function/1 -> sin/1
  Constant/1 -> Trigonometric Function/1

== system CDSC/CDSC-PLL/DSC5/DSC_Beta/2*pi*hr//n ==
  note: 2*pi*hr/n
  Constant : Constant  Value=2*pi*hr/n
  Trigonometric Function : Trigonometry  Operator=cos
  cos : Outport
  wires:
  Constant/1 -> Trigonometric Function/1
  Trigonometric Function/1 -> cos/1

== system CDSC/CDSC-PLL/DSC5/DSC_Beta/Cos 2*pi//n1 ==
  note: 2*pi*hr/n
  Constant : Constant  Value=2*pi*hr/n
  Trigonometric Function : Trigonometry
  sin : Outport
  wires:
  Constant/1 -> Trigonometric Function/1
  Trigonometric Function/1 -> sin/1

== system CDSC/CDSC-PLL/DSC5/DSC_alpha/Cos 2*pi*hr//n ==
  note: 2*pi*hr/n
  Constant : Constant  Value=2*pi*hr/n
  Trigonometric Function : Trigonometry  Operator=cos
  cos : Outport
  wires:
  Constant/1 -> Trigonometric Function/1
  Trigonometric Function/1 -> cos/1

== system CDSC/CDSC-PLL/DSC5/DSC_alpha/Cos 2*pi*hr//n1 ==
  note: 2*pi*hr/n
  Constant : Constant  Value=2*pi*hr/n
  Trigonometric Function : Trigonometry
  sin : Outport
  wires:
  Constant/1 -> Trigonometric Function/1
  Trigonometric Function/1 -> sin/1

== system CDSC/CDSC-PLL/DSC6/DSC_Beta/2*pi*hr//n ==
  note: 2*pi*hr/n
  Constant : Constant  Value=2*pi*hr/n
  Trigonometric Function : Trigonometry  Operator=cos
  cos : Outport
  wires:
  Trigonometric Function/1 -> cos/1
  Constant/1 -> Trigonometric Function/1

== system CDSC/CDSC-PLL/DSC6/DSC_Beta/Cos 2*pi//n1 ==
  note: 2*pi*hr/n
  Constant : Constant  Value=2*pi*hr/n
  Trigonometric Function : Trigonometry
  sin : Outport
  wires:
  Trigonometric Function/1 -> sin/1
  Constant/1 -> Trigonometric Function/1

== system CDSC/CDSC-PLL/DSC6/DSC_alpha/Cos 2*pi*hr//n ==
  note: 2*pi*hr/n
  Constant : Constant  Value=2*pi*hr/n
  Trigonometric Function : Trigonometry  Operator=cos
  cos : Outport
  wires:
  Trigonometric Function/1 -> cos/1
  Constant/1 -> Trigonometric Function/1

== system CDSC/CDSC-PLL/DSC6/DSC_alpha/Cos 2*pi*hr//n1 ==
  note: 2*pi*hr/n
  Constant : Constant  Value=2*pi*hr/n
  Trigonometric Function : Trigonometry
  sin : Outport
  wires:
  Trigonometric Function/1 -> sin/1
  Constant/1 -> Trigonometric Function/1

== system CDSC/CDSC-PLL/DSC8/DSC_Beta/Cos 2*pi//n ==
  note: 2*pi*hr/n
  Constant : Constant  Value=2*pi/n
  Trigonometric Function : Trigonometry  Operator=cos
  cos : Outport
  wires:
  Trigonometric Function/1 -> cos/1
  Constant/1 -> Trigonometric Function/1

== system CDSC/CDSC-PLL/DSC8/DSC_Beta/Sin 2*pi//n ==
  note: 2*pi/n
  Constant : Constant  Value=2*pi/n
  Trigonometric Function : Trigonometry
  sin : Outport
  wires:
  Trigonometric Function/1 -> sin/1
  Constant/1 -> Trigonometric Function/1

== system CDSC/CDSC-PLL/DSC8/DSC_alpha/Cos 2*pi//n ==
  note: 2*pi*hr/n
  Constant : Constant  Value=2*pi/n
  Trigonometric Function : Trigonometry  Operator=cos
  cos : Outport
  wires:
  Trigonometric Function/1 -> cos/1
  Constant/1 -> Trigonometric Function/1

== system CDSC/CDSC-PLL/DSC8/DSC_alpha/Sin 2*pi//n ==
  note: 2*pi/n
  Constant : Constant  Value=2*pi/n
  Trigonometric Function : Trigonometry
  sin : Outport
  wires:
  Trigonometric Function/1 -> sin/1
  Constant/1 -> Trigonometric Function/1
